simulink model "Acquisition_from_autosave"  (R2017a)
settings: Solver=VariableStepAuto  StartTime=0.0  StopTime=0.5  RelTol=1e-3
undefined symbols (not defined in the file): magnitude, Radix
libraries: simulink x34, commfilt2 x30, dspswit3 x12, dspmtrx3 x12, dspxfrm3 x3, simulink_extras x2, dspbuff3 x1
(part 2 of 4)

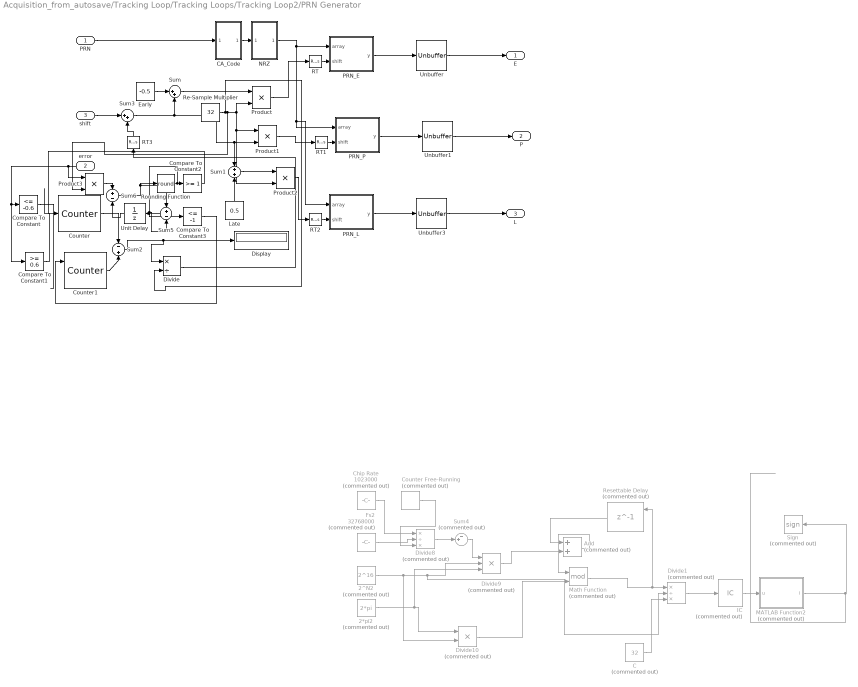
== system Acquisition_from_autosave/Tracking Loop/Tracking Loops/Tracking Loop2/PRN Generator  ==
  PRN : Inport
  error : Inport  Port=2  SampleTime=0.001
  shift : Inport  Port=3
  2*pi2 : Constant  Commented=on  Value=2*pi
  2^N2 : Constant  Commented=on  Value=2^16
  Add : Sum  Commented=on
  C : Constant  Commented=on  Value=32
  "CA_Code " : Subsystem
  Chip Rate : Constant  Commented=on  Value=1023000
  Compare To Constant : simulink/Logic and Bit Operations/Compare To Constant  relop=<=  const=-0.6  OutDataTypeStr=boolean
  Compare To Constant1 : simulink/Logic and Bit Operations/Compare To Constant  relop=>=  const=0.6  OutDataTypeStr=boolean
  Compare To Constant2 : simulink/Logic and Bit Operations/Compare To Constant  relop=>=  const=1  OutDataTypeStr=uint8
  Compare To Constant3 : simulink/Logic and Bit Operations/Compare To Constant  relop=<=  const=-1  OutDataTypeStr=uint8
  Counter : dspswit3/Counter  Direction=Up  CountEvent=Non-zero sample  CounterSize=User defined  MaxCount=255  InitialCount=0  Output=Count  HitValue=32  ResetInput=off  SamplesPerFrame=1  Ts=1  CntDtype=double  HitDtype=Logical
  Counter Free-Running : simulink/Sources/Counter Free-Running  Commented=on  NumBits=15  tsamp=1/32768000
  Counter1 : dspswit3/Counter  Direction=Up  CountEvent=Non-zero sample  CounterSize=User defined  MaxCount=255  InitialCount=0  Output=Count  HitValue=32  ResetInput=on  SamplesPerFrame=1  Ts=1  CntDtype=double  HitDtype=Logical
  Display : Display
  Divide : Product  Inputs=*/
  Divide1 : Product  Commented=on  Inputs=*/*
  Divide10 : Product  Commented=on
  Divide8 : Product  Commented=on  Inputs=*/*
  Divide9 : Product  Commented=on  Inputs=***
  Early : Constant  Value=-0.5
  Fs2 : Constant  Commented=on  Value=32768000
  IC : InitialCondition  Commented=on  Value=1023000
  Late : Constant  Value=0.5
  MATLAB Function2 : MATLAB Function  Commented=on  TreatAsAtomicUnit=on
  Math Function : Math  Commented=on  Operator=mod  SaturateOnIntegerOverflow=on
  NRZ : Subsystem
  PRN_E : MATLAB Function  TreatAsAtomicUnit=on  SystemSampleTime=0.001
  PRN_L : MATLAB Function  TreatAsAtomicUnit=on  SystemSampleTime=0.001
  PRN_P : MATLAB Function  TreatAsAtomicUnit=on  SystemSampleTime=0.001
  Product{,1..3} (4 alike) : Product
  RT : RateTransition  OutPortSampleTime=0.001
  RT1 : RateTransition  OutPortSampleTime=0.001
  RT2 : RateTransition  OutPortSampleTime=0.001
  RT3 : RateTransition
  Re-Sample Multiplier : Constant  Value=32
  Resettable Delay : Delay  Commented=on  DelayLength=1  ExternalReset=Rising  SampleTime=0.001
      settings: InputPortMap=u0,r5
  Rounding Function : Rounding  Operator=round
  Sign : Signum  Commented=on
  Sum : Sum  Inputs=|++
  Sum1 : Sum
  Sum2 : Sum  Inputs=-+
  Sum3 : Sum  Inputs=|++
  Sum4 : Sum  Commented=on  Inputs=-+|
  Sum5 : Sum  Inputs=+-
  Sum6 : Sum  Inputs=+-
  Unbuffer : Unbuffer
  Unbuffer1 : Unbuffer
  Unbuffer3 : Unbuffer
  Unit Delay : UnitDelay  SampleTime=0.001
  E : Outport
  P : Outport  Port=2
  L : Outport  Port=3
  wires:
  Product/1 -> RT/1
  PRN_E/1(y) -> Unbuffer/1
  Product2/1 -> RT2/1
  PRN_L/1(y) -> Unbuffer3/1
  Re-Sample Multiplier/1 -> Divide/2, Product3/2, Product1/1, Product2/2, Product/2
  PRN/1 -> "CA_Code "/1(In1)
  Unbuffer1/1 -> P/1
  Unbuffer3/1 -> L/1
  Early/1 -> Sum/1
  Sum/1 -> Product/1
  Sum3/1 -> Product1/2, Sum1/1, Sum/2
  Sum1/1 -> Product2/1
  PRN_P/1(y) -> Unbuffer1/1
  error/1 -> Product3/1, Compare To Constant1/1, Compare To Constant/1
  Counter/1 -> Sum2/1
  Counter1/1 -> Sum2/2
  Sum2/1 -> Divide/1, Display/1
  shift/1 -> Sum3/1
  RT/1 -> PRN_E/2(shift)
  RT1/1 -> PRN_P/2(shift)
  RT2/1 -> PRN_L/2(shift)
  Late/1 -> Sum1/2
  "CA_Code "/1(Out1) -> NRZ/1(In1)
  Unbuffer/1 -> E/1
  NRZ/1(Out1) -> PRN_E/1(array), PRN_L/1(array), PRN_P/1(array)
  Product1/1 -> RT1/1
  RT3/1 -> Sum3/2
  Compare To Constant1/1 -> ?
  Compare To Constant/1 -> ?
  MATLAB Function2/1(I) -> Sign/1
  Divide8/1 -> Sum4/2
  C/1 -> Divide1/3
  2^N2/1 -> Divide10/2, Divide1/2, Divide9/2
  Fs2/1 -> Divide8/2
  2*pi2/1 -> Divide9/3, Divide10/1
  Sum4/1 -> Divide9/1
  IC/1 -> MATLAB Function2/1(u)
  Divide10/1 -> Math Function/2
  Chip Rate/1 -> Divide8/1
  Resettable Delay/1 -> Add/1
  Divide1/1 -> IC/1
  Divide9/1 -> Add/2
  Counter Free-Running/1 -> Divide8/3
  Add/1 -> Math Function/1
  Math Function/1 -> Resettable Delay/1, Divide1/1
  Compare To Constant2/1 -> Counter/1
  Compare To Constant3/1 -> Counter1/1
  Divide/1 -> RT3/1
  Rounding Function/1 -> Sum5/2, Compare To Constant3/1, Compare To Constant2/1
  Product3/1 -> Sum6/1
  Sum5/1 -> Unit Delay/1
  Sum6/1 -> Sum5/1, Rounding Function/1
  Unit Delay/1 -> Sum6/2

== system Acquisition_from_autosave/Tracking Loop/Tracking Loops/Tracking Loop3/Carrier Filter ==
  In2 : Inport
  Add : Sum
  Constant : Constant  Value=0.001
  Constant1 : Constant  Value=-1
  Constant2 : Constant
  Constant3 : Constant  Value=-1
  Delay : Delay  DelayLength=1  InitialCondition=0  SampleTime=0.001
  Discrete FIR Filter : DiscreteFir  CoefSource=Input port  Coefficients=[2 1]  SampleTime=0.001
      settings: InputPortMap=u0,u1
  Discrete Filter : DiscreteFilter  NumeratorSource=Input port  DenominatorSource=Input port  SampleTime=0.001  a0EqualsOne=on
      settings: InputPortMap=u0,p1,p3
  Filter Parameters : Subsystem
  Product{,2..4} (4 alike) : Product
  Product1 : Product  Inputs=3
  Subsystem : Subsystem
  Sum : Sum  Inputs=|++
  Sum1 : Sum  Inputs=|++
  Sum3 : Sum  Inputs=|+-
  Sum4 : Sum  Inputs=+++
  Unit Delay : UnitDelay  SampleTime=0.001
  Unit Delay1 : UnitDelay  SampleTime=0.001
  Vector Concatenate : Concatenate
  Vector Concatenate1 : Concatenate
  Out1 : Outport
  wires:
  Product2/1 -> Sum/1
  Sum/1 -> Delay/1, Sum1/1
  Delay/1 -> Sum/2
  Product3/1 -> Sum1/2
  Unit Delay/1 -> Sum3/2
  Filter Parameters/1(K1) -> Product/2
  Filter Parameters/2(K2) -> Product1/2
  Constant/1 -> Product1/1
  Product1/1 -> Sum4/2
  Product/1 -> Sum4/1
  Sum4/1 -> Unit Delay1/1
  Unit Delay1/1 -> Sum4/3
  Subsystem/1("K2 ") -> Add/1, Product2/2
  Subsystem/2(K1) -> Product4/1, Add/2, Product3/1
  Sum3/1 -> Unit Delay/1, Product/1
  In2/1 -> Discrete Filter/1, Discrete FIR Filter/1, Product3/2, Product2/1
  ? -> Product1/3, Sum3/1
  Vector Concatenate/1 -> Discrete Filter/2, Discrete FIR Filter/2
  Constant1/1 -> Product4/2
  Product4/1 -> Vector Concatenate/2
  Add/1 -> Vector Concatenate/1
  Discrete Filter/1 -> Out1/1
  Constant2/1 -> Vector Concatenate1/1
  Constant3/1 -> Vector Concatenate1/2
  Vector Concatenate1/1 -> Discrete Filter/3

== system Acquisition_from_autosave/Tracking Loop/Tracking Loops/Tracking Loop3/Carrier Loop Discriminator  ==
  I_P : Inport
  Q_P : Inport  Port=2
  Constant : Constant  Value=2*pi
  Divide : Product  Inputs=/*
  Divide1 : Product  Inputs=*/
  IC : InitialCondition  Value=0
  IC1 : InitialCondition
  IC2 : InitialCondition
  atan : Trigonometry  Operator=atan
  theta : Outport
  wires:
  atan/1 -> Divide1/1
  Divide/1 -> atan/1
  I_P/1 -> IC1/1
  IC/1 -> theta/1
  Constant/1 -> Divide1/2
  Divide1/1 -> IC/1
  Q_P/1 -> IC2/1
  IC1/1 -> Divide/1
  IC2/1 -> Divide/2

== system Acquisition_from_autosave/Tracking Loop/Tracking Loops/Tracking Loop3/Code Filter ==
  In1 : Inport  SampleTime=0.001
  Add : Sum
  BW : Constant  Value=25
  Coeffiecients : Subsystem
  Constant : Constant  Value=2*pi
  Delay : Delay  DelayLength=1  InitialCondition=0  SampleTime=0.001
  Delay1 : Delay  DelayLength=1  InitialCondition=0  SampleTime=0.001
  Display : Display
  Display1 : Display
  Divide : Product  Inputs=*/
  Divide1 : Product  Inputs=**
  Divide2 : Product  Inputs=**
  Subtract : Sum  Inputs=-++
  ts : Constant  Value=0.001
  zeta : Constant  Value=0.7
  Out1 : Outport
  wires:
  Constant/1 -> Divide/2
  Divide/1 -> Delay/1, Divide2/1
  BW/1 -> Coeffiecients/1(BW)
  zeta/1 -> Coeffiecients/2(Zeta)
  ts/1 -> Coeffiecients/3(ts)
  Coeffiecients/1(C1) -> Add/1, Divide1/2
  Delay/1 -> Divide1/1
  Coeffiecients/2(C2) -> Add/2
  Add/1 -> Divide2/2
  Divide1/1 -> Subtract/1
  Divide2/1 -> Subtract/2
  Subtract/1 -> Out1/1, Delay1/1
  Delay1/1 -> Subtract/3
  In1/1 -> Divide/1

== system Acquisition_from_autosave/Tracking Loop/Tracking Loops/Tracking Loop3/Code Loop Discriminator ==
  I_E : Inport
  I_L : Inport  Port=2
  Q_E : Inport  Port=3
  Q_L : Inport  Port=4
  Add : Sum
  Add1 : Sum
  Add2 : Sum  Inputs=+-
  Add3 : Sum
  Display : Display
  Divide : Product  Inputs=*/
  IC : InitialCondition  Value=0
  Math Function{,2..3,5} (4 alike) : Math  Operator=magnitude^2  RndMeth=Zero  SaturateOnIntegerOverflow=on
  Sqrt : Sqrt  SaturateOnIntegerOverflow=on
  Sqrt1 : Sqrt  SaturateOnIntegerOverflow=on
  error : Outport
  wires:
  I_L/1 -> Math Function2/1
  I_E/1 -> Math Function/1
  Q_E/1 -> Math Function3/1
  Q_L/1 -> Math Function5/1
  Math Function2/1 -> Add1/1
  Math Function5/1 -> Add1/2
  Math Function/1 -> Add/1
  Math Function3/1 -> Add/2
  Add2/1 -> Divide/1
  Add3/1 -> Divide/2
  Divide/1 -> IC/1
  IC/1 -> Display/1, error/1
  Add/1 -> Sqrt/1
  Add1/1 -> Sqrt1/1
  Sqrt/1 -> Add3/1, Add2/1
  Sqrt1/1 -> Add3/2, Add2/2

== system Acquisition_from_autosave/Tracking Loop/Tracking Loops/Tracking Loop3/Controlled Carrier Generator ==
  Freq ACQ : Inport
  Phase Error : Inport  Port=2
  Freq Error : Inport  Port=3
  Clock : Clock  Commented=on
  Clock1 : Clock
  Discrete Derivative : simulink/Discrete/Discrete Derivative  gainval=1.0  ICPrevScaledInput=0.0  OutMin=[]  OutMax=[]  OutDataType=fixdt(1, 16)  OutScaling=2^-10  DoSatur=off
  Display : Display
  MATLAB Function : MATLAB Function  TreatAsAtomicUnit=on
  MATLAB Function1 : MATLAB Function  Commented=on  TreatAsAtomicUnit=on
  Sum : Sum  Inputs=++|
  "wave " : Outport
  wires:
  Clock/1 -> MATLAB Function1/2(timer)
  Freq Error/1 -> Sum/1
  Freq ACQ/1 -> Sum/2
  Sum/1 -> MATLAB Function/2(freq)
  Clock1/1 -> MATLAB Function/1(time)
  Phase Error/1 -> Discrete Derivative/1, MATLAB Function/3(phase)
  MATLAB Function/1(wave) -> "wave "/1
  Discrete Derivative/1 -> Display/1

== system Acquisition_from_autosave/Tracking Loop/Tracking Loops/Tracking Loop3/Oscillator ==
  phase error : Inport
  Acq Freq : Inport  Port=2
  2*pi2 : Constant  Value=2*pi
  2^N2 : Constant  Value=2^16
  Add : Sum
  Counter Free-Running : simulink/Sources/Counter Free-Running  NumBits=15  tsamp=1/32768000
  Divide1 : Product  Inputs=*/
  Divide10 : Product
  Divide8 : Product  Inputs=*/*
  Divide9 : Product  Inputs=***
  Fs2 : Constant  Value=32768000
  IC : InitialCondition  Value=9207000
  MATLAB Function2 : MATLAB Function  TreatAsAtomicUnit=on
  Math Function : Math  Operator=mod  SaturateOnIntegerOverflow=on
  Pulse Generator1 : DiscretePulseGenerator  PulseType=Time based  Period=0.005  PulseWidth=50
  RT2 : RateTransition
  Real-Imag to Complex2 : RealImagToComplex
  Resettable Delay : Delay  DelayLength=1  ExternalReset=Rising  SampleTime=0.001
      settings: InputPortMap=u0,r5
  Sum2 : Sum  Inputs=-+|
  Out1 : Outport
  wires:
  2*pi2/1 -> Divide9/3, Divide10/1
  Sum2/1 -> Divide9/1
  Divide8/1 -> Sum2/2
  2^N2/1 -> Divide10/2, Divide1/2, Divide9/2
  Fs2/1 -> Divide8/2
  Divide10/1 -> Math Function/2
  phase error/1 -> Sum2/1
  Acq Freq/1 -> Divide8/1
  Pulse Generator1/1 -> RT2/1
  MATLAB Function2/1(I) -> Real-Imag to Complex2/1
  MATLAB Function2/2(Q) -> Real-Imag to Complex2/2
  Divide1/1 -> IC/1
  IC/1 -> MATLAB Function2/1(u)
  Resettable Delay/1 -> Add/1
  Math Function/1 -> Resettable Delay/1, Divide1/1
  Add/1 -> Math Function/1
  Divide9/1 -> Add/2
  Real-Imag to Complex2/1 -> Out1/1
  Counter Free-Running/1 -> Divide8/3

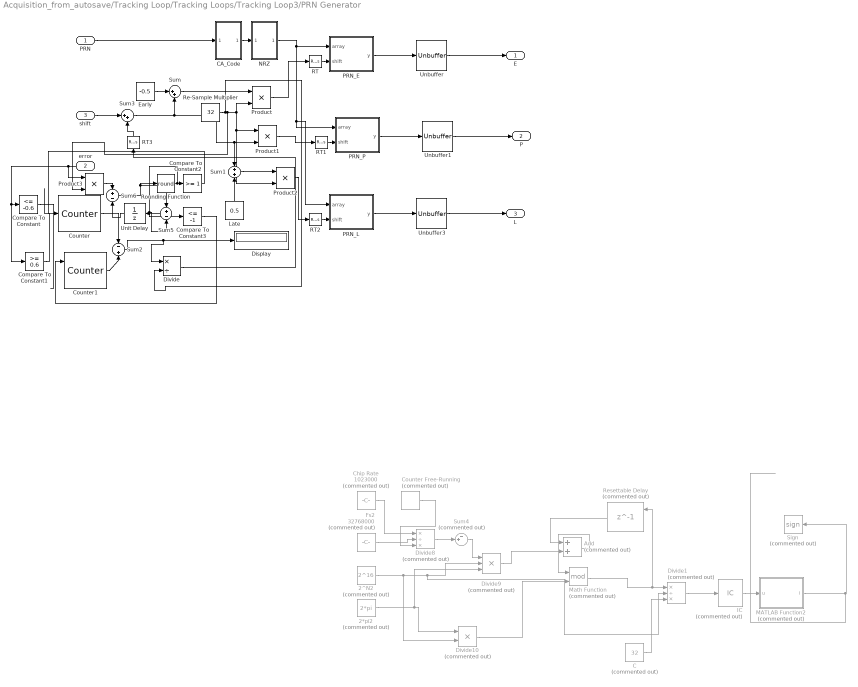
== system Acquisition_from_autosave/Tracking Loop/Tracking Loops/Tracking Loop3/PRN Generator  ==
  PRN : Inport
  error : Inport  Port=2  SampleTime=0.001
  shift : Inport  Port=3
  2*pi2 : Constant  Commented=on  Value=2*pi
  2^N2 : Constant  Commented=on  Value=2^16
  Add : Sum  Commented=on
  C : Constant  Commented=on  Value=32
  "CA_Code " : Subsystem
  Chip Rate : Constant  Commented=on  Value=1023000
  Compare To Constant : simulink/Logic and Bit Operations/Compare To Constant  relop=<=  const=-0.6  OutDataTypeStr=boolean
  Compare To Constant1 : simulink/Logic and Bit Operations/Compare To Constant  relop=>=  const=0.6  OutDataTypeStr=boolean
  Compare To Constant2 : simulink/Logic and Bit Operations/Compare To Constant  relop=>=  const=1  OutDataTypeStr=uint8
  Compare To Constant3 : simulink/Logic and Bit Operations/Compare To Constant  relop=<=  const=-1  OutDataTypeStr=uint8
  Counter : dspswit3/Counter  Direction=Up  CountEvent=Non-zero sample  CounterSize=User defined  MaxCount=255  InitialCount=0  Output=Count  HitValue=32  ResetInput=off  SamplesPerFrame=1  Ts=1  CntDtype=double  HitDtype=Logical
  Counter Free-Running : simulink/Sources/Counter Free-Running  Commented=on  NumBits=15  tsamp=1/32768000
  Counter1 : dspswit3/Counter  Direction=Up  CountEvent=Non-zero sample  CounterSize=User defined  MaxCount=255  InitialCount=0  Output=Count  HitValue=32  ResetInput=on  SamplesPerFrame=1  Ts=1  CntDtype=double  HitDtype=Logical
  Display : Display
  Divide : Product  Inputs=*/
  Divide1 : Product  Commented=on  Inputs=*/*
  Divide10 : Product  Commented=on
  Divide8 : Product  Commented=on  Inputs=*/*
  Divide9 : Product  Commented=on  Inputs=***
  Early : Constant  Value=-0.5
  Fs2 : Constant  Commented=on  Value=32768000
  IC : InitialCondition  Commented=on  Value=1023000
  Late : Constant  Value=0.5
  MATLAB Function2 : MATLAB Function  Commented=on  TreatAsAtomicUnit=on
  Math Function : Math  Commented=on  Operator=mod  SaturateOnIntegerOverflow=on
  NRZ : Subsystem
  PRN_E : MATLAB Function  TreatAsAtomicUnit=on  SystemSampleTime=0.001
  PRN_L : MATLAB Function  TreatAsAtomicUnit=on  SystemSampleTime=0.001
  PRN_P : MATLAB Function  TreatAsAtomicUnit=on  SystemSampleTime=0.001
  Product{,1..3} (4 alike) : Product
  RT : RateTransition  OutPortSampleTime=0.001
  RT1 : RateTransition  OutPortSampleTime=0.001
  RT2 : RateTransition  OutPortSampleTime=0.001
  RT3 : RateTransition
  Re-Sample Multiplier : Constant  Value=32
  Resettable Delay : Delay  Commented=on  DelayLength=1  ExternalReset=Rising  SampleTime=0.001
      settings: InputPortMap=u0,r5
  Rounding Function : Rounding  Operator=round
  Sign : Signum  Commented=on
  Sum : Sum  Inputs=|++
  Sum1 : Sum
  Sum2 : Sum  Inputs=-+
  Sum3 : Sum  Inputs=|++
  Sum4 : Sum  Commented=on  Inputs=-+|
  Sum5 : Sum  Inputs=+-
  Sum6 : Sum  Inputs=+-
  Unbuffer : Unbuffer
  Unbuffer1 : Unbuffer
  Unbuffer3 : Unbuffer
  Unit Delay : UnitDelay  SampleTime=0.001
  E : Outport
  P : Outport  Port=2
  L : Outport  Port=3
  wires:
  Product/1 -> RT/1
  PRN_E/1(y) -> Unbuffer/1
  Product2/1 -> RT2/1
  PRN_L/1(y) -> Unbuffer3/1
  Re-Sample Multiplier/1 -> Divide/2, Product3/2, Product1/1, Product2/2, Product/2
  PRN/1 -> "CA_Code "/1(In1)
  Unbuffer1/1 -> P/1
  Unbuffer3/1 -> L/1
  Early/1 -> Sum/1
  Sum/1 -> Product/1
  Sum3/1 -> Product1/2, Sum1/1, Sum/2
  Sum1/1 -> Product2/1
  PRN_P/1(y) -> Unbuffer1/1
  error/1 -> Product3/1, Compare To Constant1/1, Compare To Constant/1
  Counter/1 -> Sum2/1
  Counter1/1 -> Sum2/2
  Sum2/1 -> Divide/1, Display/1
  shift/1 -> Sum3/1
  RT/1 -> PRN_E/2(shift)
  RT1/1 -> PRN_P/2(shift)
  RT2/1 -> PRN_L/2(shift)
  Late/1 -> Sum1/2
  "CA_Code "/1(Out1) -> NRZ/1(In1)
  Unbuffer/1 -> E/1
  NRZ/1(Out1) -> PRN_E/1(array), PRN_L/1(array), PRN_P/1(array)
  Product1/1 -> RT1/1
  RT3/1 -> Sum3/2
  Compare To Constant1/1 -> ?
  Compare To Constant/1 -> ?
  MATLAB Function2/1(I) -> Sign/1
  Divide8/1 -> Sum4/2
  C/1 -> Divide1/3
  2^N2/1 -> Divide10/2, Divide1/2, Divide9/2
  Fs2/1 -> Divide8/2
  2*pi2/1 -> Divide9/3, Divide10/1
  Sum4/1 -> Divide9/1
  IC/1 -> MATLAB Function2/1(u)
  Divide10/1 -> Math Function/2
  Chip Rate/1 -> Divide8/1
  Resettable Delay/1 -> Add/1
  Divide1/1 -> IC/1
  Divide9/1 -> Add/2
  Counter Free-Running/1 -> Divide8/3
  Add/1 -> Math Function/1
  Math Function/1 -> Resettable Delay/1, Divide1/1
  Compare To Constant2/1 -> Counter/1
  Compare To Constant3/1 -> Counter1/1
  Divide/1 -> RT3/1
  Rounding Function/1 -> Sum5/2, Compare To Constant3/1, Compare To Constant2/1
  Product3/1 -> Sum6/1
  Sum5/1 -> Unit Delay/1
  Sum6/1 -> Sum5/1, Rounding Function/1
  Unit Delay/1 -> Sum6/2

== system Acquisition_from_autosave/Tracking Loop/Tracking Loops/Tracking Loop4/Carrier Filter ==
  In2 : Inport
  Add : Sum
  Constant : Constant  Value=0.001
  Constant1 : Constant  Value=-1
  Constant2 : Constant
  Constant3 : Constant  Value=-1
  Delay : Delay  DelayLength=1  InitialCondition=0  SampleTime=0.001
  Discrete FIR Filter : DiscreteFir  CoefSource=Input port  Coefficients=[2 1]  SampleTime=0.001
      settings: InputPortMap=u0,u1
  Discrete Filter : DiscreteFilter  NumeratorSource=Input port  DenominatorSource=Input port  SampleTime=0.001  a0EqualsOne=on
      settings: InputPortMap=u0,p1,p3
  Filter Parameters : Subsystem
  Product{,2..4} (4 alike) : Product
  Product1 : Product  Inputs=3
  Subsystem : Subsystem
  Sum : Sum  Inputs=|++
  Sum1 : Sum  Inputs=|++
  Sum3 : Sum  Inputs=|+-
  Sum4 : Sum  Inputs=+++
  Unit Delay : UnitDelay  SampleTime=0.001
  Unit Delay1 : UnitDelay  SampleTime=0.001
  Vector Concatenate : Concatenate
  Vector Concatenate1 : Concatenate
  Out1 : Outport
  wires:
  Product2/1 -> Sum/1
  Sum/1 -> Delay/1, Sum1/1
  Delay/1 -> Sum/2
  Product3/1 -> Sum1/2
  Unit Delay/1 -> Sum3/2
  Filter Parameters/1(K1) -> Product/2
  Filter Parameters/2(K2) -> Product1/2
  Constant/1 -> Product1/1
  Product1/1 -> Sum4/2
  Product/1 -> Sum4/1
  Sum4/1 -> Unit Delay1/1
  Unit Delay1/1 -> Sum4/3
  Subsystem/1("K2 ") -> Add/1, Product2/2
  Subsystem/2(K1) -> Product4/1, Add/2, Product3/1
  Sum3/1 -> Unit Delay/1, Product/1
  In2/1 -> Discrete Filter/1, Discrete FIR Filter/1, Product3/2, Product2/1
  ? -> Product1/3, Sum3/1
  Vector Concatenate/1 -> Discrete Filter/2, Discrete FIR Filter/2
  Constant1/1 -> Product4/2
  Product4/1 -> Vector Concatenate/2
  Add/1 -> Vector Concatenate/1
  Discrete Filter/1 -> Out1/1
  Constant2/1 -> Vector Concatenate1/1
  Constant3/1 -> Vector Concatenate1/2
  Vector Concatenate1/1 -> Discrete Filter/3

== system Acquisition_from_autosave/Tracking Loop/Tracking Loops/Tracking Loop4/Carrier Loop Discriminator  ==
  I_P : Inport
  Q_P : Inport  Port=2
  Constant : Constant  Value=2*pi
  Divide : Product  Inputs=/*
  Divide1 : Product  Inputs=*/
  IC : InitialCondition  Value=0
  IC1 : InitialCondition
  IC2 : InitialCondition
  atan : Trigonometry  Operator=atan
  theta : Outport
  wires:
  atan/1 -> Divide1/1
  Divide/1 -> atan/1
  I_P/1 -> IC1/1
  IC/1 -> theta/1
  Constant/1 -> Divide1/2
  Divide1/1 -> IC/1
  Q_P/1 -> IC2/1
  IC1/1 -> Divide/1
  IC2/1 -> Divide/2

== system Acquisition_from_autosave/Tracking Loop/Tracking Loops/Tracking Loop4/Code Filter ==
  In1 : Inport  SampleTime=0.001
  Add : Sum
  BW : Constant  Value=25
  Coeffiecients : Subsystem
  Constant : Constant  Value=2*pi
  Delay : Delay  DelayLength=1  InitialCondition=0  SampleTime=0.001
  Delay1 : Delay  DelayLength=1  InitialCondition=0  SampleTime=0.001
  Display : Display
  Display1 : Display
  Divide : Product  Inputs=*/
  Divide1 : Product  Inputs=**
  Divide2 : Product  Inputs=**
  Subtract : Sum  Inputs=-++
  ts : Constant  Value=0.001
  zeta : Constant  Value=0.7
  Out1 : Outport
  wires:
  Constant/1 -> Divide/2
  Divide/1 -> Delay/1, Divide2/1
  BW/1 -> Coeffiecients/1(BW)
  zeta/1 -> Coeffiecients/2(Zeta)
  ts/1 -> Coeffiecients/3(ts)
  Coeffiecients/1(C1) -> Add/1, Divide1/2
  Delay/1 -> Divide1/1
  Coeffiecients/2(C2) -> Add/2
  Add/1 -> Divide2/2
  Divide1/1 -> Subtract/1
  Divide2/1 -> Subtract/2
  Subtract/1 -> Out1/1, Delay1/1
  Delay1/1 -> Subtract/3
  In1/1 -> Divide/1

== system Acquisition_from_autosave/Tracking Loop/Tracking Loops/Tracking Loop4/Code Loop Discriminator ==
  I_E : Inport
  I_L : Inport  Port=2
  Q_E : Inport  Port=3
  Q_L : Inport  Port=4
  Add : Sum
  Add1 : Sum
  Add2 : Sum  Inputs=+-
  Add3 : Sum
  Display : Display
  Divide : Product  Inputs=*/
  IC : InitialCondition  Value=0
  Math Function{,2..3,5} (4 alike) : Math  Operator=magnitude^2  RndMeth=Zero  SaturateOnIntegerOverflow=on
  Sqrt : Sqrt  SaturateOnIntegerOverflow=on
  Sqrt1 : Sqrt  SaturateOnIntegerOverflow=on
  error : Outport
  wires:
  I_L/1 -> Math Function2/1
  I_E/1 -> Math Function/1
  Q_E/1 -> Math Function3/1
  Q_L/1 -> Math Function5/1
  Math Function2/1 -> Add1/1
  Math Function5/1 -> Add1/2
  Math Function/1 -> Add/1
  Math Function3/1 -> Add/2
  Add2/1 -> Divide/1
  Add3/1 -> Divide/2
  Divide/1 -> IC/1
  IC/1 -> Display/1, error/1
  Add/1 -> Sqrt/1
  Add1/1 -> Sqrt1/1
  Sqrt/1 -> Add3/1, Add2/1
  Sqrt1/1 -> Add3/2, Add2/2

== system Acquisition_from_autosave/Tracking Loop/Tracking Loops/Tracking Loop4/Controlled Carrier Generator ==
  Freq ACQ : Inport
  Phase Error : Inport  Port=2
  Freq Error : Inport  Port=3
  Clock : Clock  Commented=on
  Clock1 : Clock
  Discrete Derivative : simulink/Discrete/Discrete Derivative  gainval=1.0  ICPrevScaledInput=0.0  OutMin=[]  OutMax=[]  OutDataType=fixdt(1, 16)  OutScaling=2^-10  DoSatur=off
  Display : Display
  MATLAB Function : MATLAB Function  TreatAsAtomicUnit=on
  MATLAB Function1 : MATLAB Function  Commented=on  TreatAsAtomicUnit=on
  Sum : Sum  Inputs=++|
  "wave " : Outport
  wires:
  Clock/1 -> MATLAB Function1/2(timer)
  Freq Error/1 -> Sum/1
  Freq ACQ/1 -> Sum/2
  Sum/1 -> MATLAB Function/2(freq)
  Clock1/1 -> MATLAB Function/1(time)
  Phase Error/1 -> Discrete Derivative/1, MATLAB Function/3(phase)
  MATLAB Function/1(wave) -> "wave "/1
  Discrete Derivative/1 -> Display/1

== system Acquisition_from_autosave/Tracking Loop/Tracking Loops/Tracking Loop4/Oscillator ==
  phase error : Inport
  Acq Freq : Inport  Port=2
  2*pi2 : Constant  Value=2*pi
  2^N2 : Constant  Value=2^16
  Add : Sum
  Counter Free-Running : simulink/Sources/Counter Free-Running  NumBits=15  tsamp=1/32768000
  Divide1 : Product  Inputs=*/
  Divide10 : Product
  Divide8 : Product  Inputs=*/*
  Divide9 : Product  Inputs=***
  Fs2 : Constant  Value=32768000
  IC : InitialCondition  Value=9207000
  MATLAB Function2 : MATLAB Function  TreatAsAtomicUnit=on
  Math Function : Math  Operator=mod  SaturateOnIntegerOverflow=on
  Pulse Generator1 : DiscretePulseGenerator  PulseType=Time based  Period=0.005  PulseWidth=50
  RT2 : RateTransition
  Real-Imag to Complex2 : RealImagToComplex
  Resettable Delay : Delay  DelayLength=1  ExternalReset=Rising  SampleTime=0.001
      settings: InputPortMap=u0,r5
  Sum2 : Sum  Inputs=-+|
  Out1 : Outport
  wires:
  2*pi2/1 -> Divide9/3, Divide10/1
  Sum2/1 -> Divide9/1
  Divide8/1 -> Sum2/2
  2^N2/1 -> Divide10/2, Divide1/2, Divide9/2
  Fs2/1 -> Divide8/2
  Divide10/1 -> Math Function/2
  phase error/1 -> Sum2/1
  Acq Freq/1 -> Divide8/1
  Pulse Generator1/1 -> RT2/1
  MATLAB Function2/1(I) -> Real-Imag to Complex2/1
  MATLAB Function2/2(Q) -> Real-Imag to Complex2/2
  Divide1/1 -> IC/1
  IC/1 -> MATLAB Function2/1(u)
  Resettable Delay/1 -> Add/1
  Math Function/1 -> Resettable Delay/1, Divide1/1
  Add/1 -> Math Function/1
  Divide9/1 -> Add/2
  Real-Imag to Complex2/1 -> Out1/1
  Counter Free-Running/1 -> Divide8/3

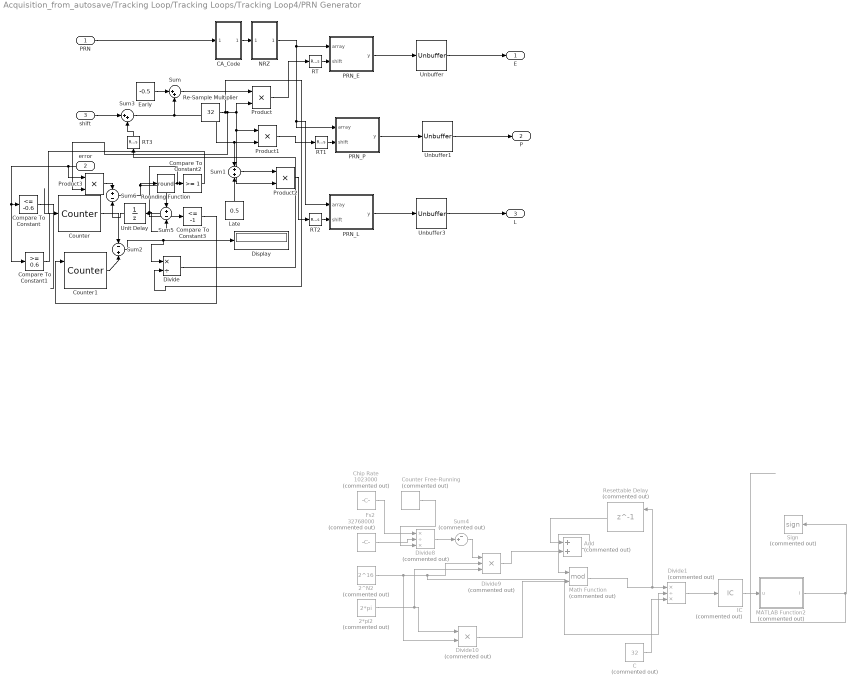
== system Acquisition_from_autosave/Tracking Loop/Tracking Loops/Tracking Loop4/PRN Generator  ==
  PRN : Inport
  error : Inport  Port=2  SampleTime=0.001
  shift : Inport  Port=3
  2*pi2 : Constant  Commented=on  Value=2*pi
  2^N2 : Constant  Commented=on  Value=2^16
  Add : Sum  Commented=on
  C : Constant  Commented=on  Value=32
  "CA_Code " : Subsystem
  Chip Rate : Constant  Commented=on  Value=1023000
  Compare To Constant : simulink/Logic and Bit Operations/Compare To Constant  relop=<=  const=-0.6  OutDataTypeStr=boolean
  Compare To Constant1 : simulink/Logic and Bit Operations/Compare To Constant  relop=>=  const=0.6  OutDataTypeStr=boolean
  Compare To Constant2 : simulink/Logic and Bit Operations/Compare To Constant  relop=>=  const=1  OutDataTypeStr=uint8
  Compare To Constant3 : simulink/Logic and Bit Operations/Compare To Constant  relop=<=  const=-1  OutDataTypeStr=uint8
  Counter : dspswit3/Counter  Direction=Up  CountEvent=Non-zero sample  CounterSize=User defined  MaxCount=255  InitialCount=0  Output=Count  HitValue=32  ResetInput=off  SamplesPerFrame=1  Ts=1  CntDtype=double  HitDtype=Logical
  Counter Free-Running : simulink/Sources/Counter Free-Running  Commented=on  NumBits=15  tsamp=1/32768000
  Counter1 : dspswit3/Counter  Direction=Up  CountEvent=Non-zero sample  CounterSize=User defined  MaxCount=255  InitialCount=0  Output=Count  HitValue=32  ResetInput=on  SamplesPerFrame=1  Ts=1  CntDtype=double  HitDtype=Logical
  Display : Display
  Divide : Product  Inputs=*/
  Divide1 : Product  Commented=on  Inputs=*/*
  Divide10 : Product  Commented=on
  Divide8 : Product  Commented=on  Inputs=*/*
  Divide9 : Product  Commented=on  Inputs=***
  Early : Constant  Value=-0.5
  Fs2 : Constant  Commented=on  Value=32768000
  IC : InitialCondition  Commented=on  Value=1023000
  Late : Constant  Value=0.5
  MATLAB Function2 : MATLAB Function  Commented=on  TreatAsAtomicUnit=on
  Math Function : Math  Commented=on  Operator=mod  SaturateOnIntegerOverflow=on
  NRZ : Subsystem
  PRN_E : MATLAB Function  TreatAsAtomicUnit=on  SystemSampleTime=0.001
  PRN_L : MATLAB Function  TreatAsAtomicUnit=on  SystemSampleTime=0.001
  PRN_P : MATLAB Function  TreatAsAtomicUnit=on  SystemSampleTime=0.001
  Product{,1..3} (4 alike) : Product
  RT : RateTransition  OutPortSampleTime=0.001
  RT1 : RateTransition  OutPortSampleTime=0.001
  RT2 : RateTransition  OutPortSampleTime=0.001
  RT3 : RateTransition
  Re-Sample Multiplier : Constant  Value=32
  Resettable Delay : Delay  Commented=on  DelayLength=1  ExternalReset=Rising  SampleTime=0.001
      settings: InputPortMap=u0,r5
  Rounding Function : Rounding  Operator=round
  Sign : Signum  Commented=on
  Sum : Sum  Inputs=|++
  Sum1 : Sum
  Sum2 : Sum  Inputs=-+
  Sum3 : Sum  Inputs=|++
  Sum4 : Sum  Commented=on  Inputs=-+|
  Sum5 : Sum  Inputs=+-
  Sum6 : Sum  Inputs=+-
  Unbuffer : Unbuffer
  Unbuffer1 : Unbuffer
  Unbuffer3 : Unbuffer
  Unit Delay : UnitDelay  SampleTime=0.001
  E : Outport
  P : Outport  Port=2
  L : Outport  Port=3
  wires:
  Product/1 -> RT/1
  PRN_E/1(y) -> Unbuffer/1
  Product2/1 -> RT2/1
  PRN_L/1(y) -> Unbuffer3/1
  Re-Sample Multiplier/1 -> Divide/2, Product3/2, Product1/1, Product2/2, Product/2
  PRN/1 -> "CA_Code "/1(In1)
  Unbuffer1/1 -> P/1
  Unbuffer3/1 -> L/1
  Early/1 -> Sum/1
  Sum/1 -> Product/1
  Sum3/1 -> Product1/2, Sum1/1, Sum/2
  Sum1/1 -> Product2/1
  PRN_P/1(y) -> Unbuffer1/1
  error/1 -> Product3/1, Compare To Constant1/1, Compare To Constant/1
  Counter/1 -> Sum2/1
  Counter1/1 -> Sum2/2
  Sum2/1 -> Divide/1, Display/1
  shift/1 -> Sum3/1
  RT/1 -> PRN_E/2(shift)
  RT1/1 -> PRN_P/2(shift)
  RT2/1 -> PRN_L/2(shift)
  Late/1 -> Sum1/2
  "CA_Code "/1(Out1) -> NRZ/1(In1)
  Unbuffer/1 -> E/1
  NRZ/1(Out1) -> PRN_E/1(array), PRN_L/1(array), PRN_P/1(array)
  Product1/1 -> RT1/1
  RT3/1 -> Sum3/2
  Compare To Constant1/1 -> ?
  Compare To Constant/1 -> ?
  MATLAB Function2/1(I) -> Sign/1
  Divide8/1 -> Sum4/2
  C/1 -> Divide1/3
  2^N2/1 -> Divide10/2, Divide1/2, Divide9/2
  Fs2/1 -> Divide8/2
  2*pi2/1 -> Divide9/3, Divide10/1
  Sum4/1 -> Divide9/1
  IC/1 -> MATLAB Function2/1(u)
  Divide10/1 -> Math Function/2
  Chip Rate/1 -> Divide8/1
  Resettable Delay/1 -> Add/1
  Divide1/1 -> IC/1
  Divide9/1 -> Add/2
  Counter Free-Running/1 -> Divide8/3
  Add/1 -> Math Function/1
  Math Function/1 -> Resettable Delay/1, Divide1/1
  Compare To Constant2/1 -> Counter/1
  Compare To Constant3/1 -> Counter1/1
  Divide/1 -> RT3/1
  Rounding Function/1 -> Sum5/2, Compare To Constant3/1, Compare To Constant2/1
  Product3/1 -> Sum6/1
  Sum5/1 -> Unit Delay/1
  Sum6/1 -> Sum5/1, Rounding Function/1
  Unit Delay/1 -> Sum6/2

== system Acquisition_from_autosave/Tracking Loop/Tracking Loops/Tracking Loop5/Carrier Filter ==
  In2 : Inport
  Add : Sum
  Constant : Constant  Value=0.001
  Constant1 : Constant  Value=-1
  Constant2 : Constant
  Constant3 : Constant  Value=-1
  Delay : Delay  DelayLength=1  InitialCondition=0  SampleTime=0.001
  Discrete FIR Filter : DiscreteFir  CoefSource=Input port  Coefficients=[2 1]  SampleTime=0.001
      settings: InputPortMap=u0,u1
  Discrete Filter : DiscreteFilter  NumeratorSource=Input port  DenominatorSource=Input port  SampleTime=0.001  a0EqualsOne=on
      settings: InputPortMap=u0,p1,p3
  Filter Parameters : Subsystem
  Product{,2..4} (4 alike) : Product
  Product1 : Product  Inputs=3
  Subsystem : Subsystem
  Sum : Sum  Inputs=|++
  Sum1 : Sum  Inputs=|++
  Sum3 : Sum  Inputs=|+-
  Sum4 : Sum  Inputs=+++
  Unit Delay : UnitDelay  SampleTime=0.001
  Unit Delay1 : UnitDelay  SampleTime=0.001
  Vector Concatenate : Concatenate
  Vector Concatenate1 : Concatenate
  Out1 : Outport
  wires:
  Product2/1 -> Sum/1
  Sum/1 -> Delay/1, Sum1/1
  Delay/1 -> Sum/2
  Product3/1 -> Sum1/2
  Unit Delay/1 -> Sum3/2
  Filter Parameters/1(K1) -> Product/2
  Filter Parameters/2(K2) -> Product1/2
  Constant/1 -> Product1/1
  Product1/1 -> Sum4/2
  Product/1 -> Sum4/1
  Sum4/1 -> Unit Delay1/1
  Unit Delay1/1 -> Sum4/3
  Subsystem/1("K2 ") -> Add/1, Product2/2
  Subsystem/2(K1) -> Product4/1, Add/2, Product3/1
  Sum3/1 -> Unit Delay/1, Product/1
  In2/1 -> Discrete Filter/1, Discrete FIR Filter/1, Product3/2, Product2/1
  ? -> Product1/3, Sum3/1
  Vector Concatenate/1 -> Discrete Filter/2, Discrete FIR Filter/2
  Constant1/1 -> Product4/2
  Product4/1 -> Vector Concatenate/2
  Add/1 -> Vector Concatenate/1
  Discrete Filter/1 -> Out1/1
  Constant2/1 -> Vector Concatenate1/1
  Constant3/1 -> Vector Concatenate1/2
  Vector Concatenate1/1 -> Discrete Filter/3

== system Acquisition_from_autosave/Tracking Loop/Tracking Loops/Tracking Loop5/Carrier Loop Discriminator  ==
  I_P : Inport
  Q_P : Inport  Port=2
  Constant : Constant  Value=2*pi
  Divide : Product  Inputs=/*
  Divide1 : Product  Inputs=*/
  IC : InitialCondition  Value=0
  IC1 : InitialCondition
  IC2 : InitialCondition
  atan : Trigonometry  Operator=atan
  theta : Outport
  wires:
  atan/1 -> Divide1/1
  Divide/1 -> atan/1
  I_P/1 -> IC1/1
  IC/1 -> theta/1
  Constant/1 -> Divide1/2
  Divide1/1 -> IC/1
  Q_P/1 -> IC2/1
  IC1/1 -> Divide/1
  IC2/1 -> Divide/2

== system Acquisition_from_autosave/Tracking Loop/Tracking Loops/Tracking Loop5/Code Filter ==
  In1 : Inport  SampleTime=0.001
  Add : Sum
  BW : Constant  Value=25
  Coeffiecients : Subsystem
  Constant : Constant  Value=2*pi
  Delay : Delay  DelayLength=1  InitialCondition=0  SampleTime=0.001
  Delay1 : Delay  DelayLength=1  InitialCondition=0  SampleTime=0.001
  Display : Display
  Display1 : Display
  Divide : Product  Inputs=*/
  Divide1 : Product  Inputs=**
  Divide2 : Product  Inputs=**
  Subtract : Sum  Inputs=-++
  ts : Constant  Value=0.001
  zeta : Constant  Value=0.7
  Out1 : Outport
  wires:
  Constant/1 -> Divide/2
  Divide/1 -> Delay/1, Divide2/1
  BW/1 -> Coeffiecients/1(BW)
  zeta/1 -> Coeffiecients/2(Zeta)
  ts/1 -> Coeffiecients/3(ts)
  Coeffiecients/1(C1) -> Add/1, Divide1/2
  Delay/1 -> Divide1/1
  Coeffiecients/2(C2) -> Add/2
  Add/1 -> Divide2/2
  Divide1/1 -> Subtract/1
  Divide2/1 -> Subtract/2
  Subtract/1 -> Out1/1, Delay1/1
  Delay1/1 -> Subtract/3
  In1/1 -> Divide/1

== system Acquisition_from_autosave/Tracking Loop/Tracking Loops/Tracking Loop5/Code Loop Discriminator ==
  I_E : Inport
  I_L : Inport  Port=2
  Q_E : Inport  Port=3
  Q_L : Inport  Port=4
  Add : Sum
  Add1 : Sum
  Add2 : Sum  Inputs=+-
  Add3 : Sum
  Display : Display
  Divide : Product  Inputs=*/
  IC : InitialCondition  Value=0
  Math Function{,2..3,5} (4 alike) : Math  Operator=magnitude^2  RndMeth=Zero  SaturateOnIntegerOverflow=on
  Sqrt : Sqrt  SaturateOnIntegerOverflow=on
  Sqrt1 : Sqrt  SaturateOnIntegerOverflow=on
  error : Outport
  wires:
  I_L/1 -> Math Function2/1
  I_E/1 -> Math Function/1
  Q_E/1 -> Math Function3/1
  Q_L/1 -> Math Function5/1
  Math Function2/1 -> Add1/1
  Math Function5/1 -> Add1/2
  Math Function/1 -> Add/1
  Math Function3/1 -> Add/2
  Add2/1 -> Divide/1
  Add3/1 -> Divide/2
  Divide/1 -> IC/1
  IC/1 -> Display/1, error/1
  Add/1 -> Sqrt/1
  Add1/1 -> Sqrt1/1
  Sqrt/1 -> Add3/1, Add2/1
  Sqrt1/1 -> Add3/2, Add2/2

== system Acquisition_from_autosave/Tracking Loop/Tracking Loops/Tracking Loop5/Controlled Carrier Generator ==
  Freq ACQ : Inport
  Phase Error : Inport  Port=2
  Freq Error : Inport  Port=3
  Clock : Clock  Commented=on
  Clock1 : Clock
  Discrete Derivative : simulink/Discrete/Discrete Derivative  gainval=1.0  ICPrevScaledInput=0.0  OutMin=[]  OutMax=[]  OutDataType=fixdt(1, 16)  OutScaling=2^-10  DoSatur=off
  Display : Display
  MATLAB Function : MATLAB Function  TreatAsAtomicUnit=on
  MATLAB Function1 : MATLAB Function  Commented=on  TreatAsAtomicUnit=on
  Sum : Sum  Inputs=++|
  "wave " : Outport
  wires:
  Clock/1 -> MATLAB Function1/2(timer)
  Freq Error/1 -> Sum/1
  Freq ACQ/1 -> Sum/2
  Sum/1 -> MATLAB Function/2(freq)
  Clock1/1 -> MATLAB Function/1(time)
  Phase Error/1 -> Discrete Derivative/1, MATLAB Function/3(phase)
  MATLAB Function/1(wave) -> "wave "/1
  Discrete Derivative/1 -> Display/1

== system Acquisition_from_autosave/Tracking Loop/Tracking Loops/Tracking Loop5/Oscillator ==
  phase error : Inport
  Acq Freq : Inport  Port=2
  2*pi2 : Constant  Value=2*pi
  2^N2 : Constant  Value=2^16
  Add : Sum
  Counter Free-Running : simulink/Sources/Counter Free-Running  NumBits=15  tsamp=1/32768000
  Divide1 : Product  Inputs=*/
  Divide10 : Product
  Divide8 : Product  Inputs=*/*
  Divide9 : Product  Inputs=***
  Fs2 : Constant  Value=32768000
  IC : InitialCondition  Value=9207000
  MATLAB Function2 : MATLAB Function  TreatAsAtomicUnit=on
  Math Function : Math  Operator=mod  SaturateOnIntegerOverflow=on
  Pulse Generator1 : DiscretePulseGenerator  PulseType=Time based  Period=0.005  PulseWidth=50
  RT2 : RateTransition
  Real-Imag to Complex2 : RealImagToComplex
  Resettable Delay : Delay  DelayLength=1  ExternalReset=Rising  SampleTime=0.001
      settings: InputPortMap=u0,r5
  Sum2 : Sum  Inputs=-+|
  Out1 : Outport
  wires:
  2*pi2/1 -> Divide9/3, Divide10/1
  Sum2/1 -> Divide9/1
  Divide8/1 -> Sum2/2
  2^N2/1 -> Divide10/2, Divide1/2, Divide9/2
  Fs2/1 -> Divide8/2
  Divide10/1 -> Math Function/2
  phase error/1 -> Sum2/1
  Acq Freq/1 -> Divide8/1
  Pulse Generator1/1 -> RT2/1
  MATLAB Function2/1(I) -> Real-Imag to Complex2/1
  MATLAB Function2/2(Q) -> Real-Imag to Complex2/2
  Divide1/1 -> IC/1
  IC/1 -> MATLAB Function2/1(u)
  Resettable Delay/1 -> Add/1
  Math Function/1 -> Resettable Delay/1, Divide1/1
  Add/1 -> Math Function/1
  Divide9/1 -> Add/2
  Real-Imag to Complex2/1 -> Out1/1
  Counter Free-Running/1 -> Divide8/3

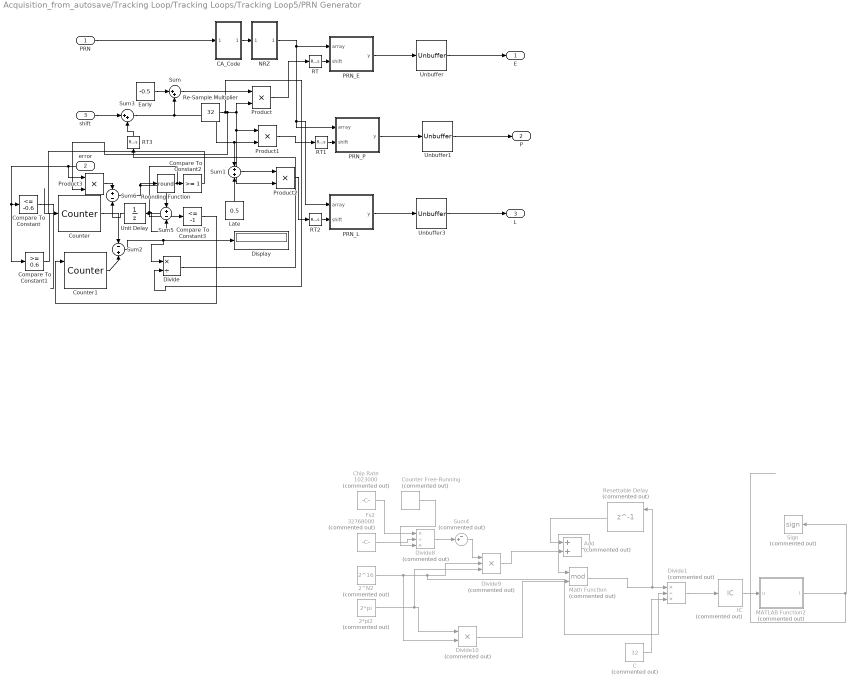
== system Acquisition_from_autosave/Tracking Loop/Tracking Loops/Tracking Loop5/PRN Generator  ==
  PRN : Inport
  error : Inport  Port=2  SampleTime=0.001
  shift : Inport  Port=3
  2*pi2 : Constant  Commented=on  Value=2*pi
  2^N2 : Constant  Commented=on  Value=2^16
  Add : Sum  Commented=on
  C : Constant  Commented=on  Value=32
  "CA_Code " : Subsystem
  Chip Rate : Constant  Commented=on  Value=1023000
  Compare To Constant : simulink/Logic and Bit Operations/Compare To Constant  relop=<=  const=-0.6  OutDataTypeStr=boolean
  Compare To Constant1 : simulink/Logic and Bit Operations/Compare To Constant  relop=>=  const=0.6  OutDataTypeStr=boolean
  Compare To Constant2 : simulink/Logic and Bit Operations/Compare To Constant  relop=>=  const=1  OutDataTypeStr=uint8
  Compare To Constant3 : simulink/Logic and Bit Operations/Compare To Constant  relop=<=  const=-1  OutDataTypeStr=uint8
  Counter : dspswit3/Counter  Direction=Up  CountEvent=Non-zero sample  CounterSize=User defined  MaxCount=255  InitialCount=0  Output=Count  HitValue=32  ResetInput=off  SamplesPerFrame=1  Ts=1  CntDtype=double  HitDtype=Logical
  Counter Free-Running : simulink/Sources/Counter Free-Running  Commented=on  NumBits=15  tsamp=1/32768000
  Counter1 : dspswit3/Counter  Direction=Up  CountEvent=Non-zero sample  CounterSize=User defined  MaxCount=255  InitialCount=0  Output=Count  HitValue=32  ResetInput=on  SamplesPerFrame=1  Ts=1  CntDtype=double  HitDtype=Logical
  Display : Display
  Divide : Product  Inputs=*/
  Divide1 : Product  Commented=on  Inputs=*/*
  Divide10 : Product  Commented=on
  Divide8 : Product  Commented=on  Inputs=*/*
  Divide9 : Product  Commented=on  Inputs=***
  Early : Constant  Value=-0.5
  Fs2 : Constant  Commented=on  Value=32768000
  IC : InitialCondition  Commented=on  Value=1023000
  Late : Constant  Value=0.5
  MATLAB Function2 : MATLAB Function  Commented=on  TreatAsAtomicUnit=on
  Math Function : Math  Commented=on  Operator=mod  SaturateOnIntegerOverflow=on
  NRZ : Subsystem
  PRN_E : MATLAB Function  TreatAsAtomicUnit=on  SystemSampleTime=0.001
  PRN_L : MATLAB Function  TreatAsAtomicUnit=on  SystemSampleTime=0.001
  PRN_P : MATLAB Function  TreatAsAtomicUnit=on  SystemSampleTime=0.001
  Product{,1..3} (4 alike) : Product
  RT : RateTransition  OutPortSampleTime=0.001
  RT1 : RateTransition  OutPortSampleTime=0.001
  RT2 : RateTransition  OutPortSampleTime=0.001
  RT3 : RateTransition
  Re-Sample Multiplier : Constant  Value=32
  Resettable Delay : Delay  Commented=on  DelayLength=1  ExternalReset=Rising  SampleTime=0.001
      settings: InputPortMap=u0,r5
  Rounding Function : Rounding  Operator=round
  Sign : Signum  Commented=on
  Sum : Sum  Inputs=|++
  Sum1 : Sum
  Sum2 : Sum  Inputs=-+
  Sum3 : Sum  Inputs=|++
  Sum4 : Sum  Commented=on  Inputs=-+|
  Sum5 : Sum  Inputs=+-
  Sum6 : Sum  Inputs=+-
  Unbuffer : Unbuffer
  Unbuffer1 : Unbuffer
  Unbuffer3 : Unbuffer
  Unit Delay : UnitDelay  SampleTime=0.001
  E : Outport
  P : Outport  Port=2
  L : Outport  Port=3
  wires:
  Product/1 -> RT/1
  PRN_E/1(y) -> Unbuffer/1
  Product2/1 -> RT2/1
  PRN_L/1(y) -> Unbuffer3/1
  Re-Sample Multiplier/1 -> Divide/2, Product3/2, Product1/1, Product2/2, Product/2
  PRN/1 -> "CA_Code "/1(In1)
  Unbuffer1/1 -> P/1
  Unbuffer3/1 -> L/1
  Early/1 -> Sum/1
  Sum/1 -> Product/1
  Sum3/1 -> Product1/2, Sum1/1, Sum/2
  Sum1/1 -> Product2/1
  PRN_P/1(y) -> Unbuffer1/1
  error/1 -> Product3/1, Compare To Constant1/1, Compare To Constant/1
  Counter/1 -> Sum2/1
  Counter1/1 -> Sum2/2
  Sum2/1 -> Divide/1, Display/1
  shift/1 -> Sum3/1
  RT/1 -> PRN_E/2(shift)
  RT1/1 -> PRN_P/2(shift)
  RT2/1 -> PRN_L/2(shift)
  Late/1 -> Sum1/2
  "CA_Code "/1(Out1) -> NRZ/1(In1)
  Unbuffer/1 -> E/1
  NRZ/1(Out1) -> PRN_E/1(array), PRN_L/1(array), PRN_P/1(array)
  Product1/1 -> RT1/1
  RT3/1 -> Sum3/2
  Compare To Constant1/1 -> ?
  Compare To Constant/1 -> ?
  MATLAB Function2/1(I) -> Sign/1
  Divide8/1 -> Sum4/2
  C/1 -> Divide1/3
  2^N2/1 -> Divide10/2, Divide1/2, Divide9/2
  Fs2/1 -> Divide8/2
  2*pi2/1 -> Divide9/3, Divide10/1
  Sum4/1 -> Divide9/1
  IC/1 -> MATLAB Function2/1(u)
  Divide10/1 -> Math Function/2
  Chip Rate/1 -> Divide8/1
  Resettable Delay/1 -> Add/1
  Divide1/1 -> IC/1
  Divide9/1 -> Add/2
  Counter Free-Running/1 -> Divide8/3
  Add/1 -> Math Function/1
  Math Function/1 -> Resettable Delay/1, Divide1/1
  Compare To Constant2/1 -> Counter/1
  Compare To Constant3/1 -> Counter1/1
  Divide/1 -> RT3/1
  Rounding Function/1 -> Sum5/2, Compare To Constant3/1, Compare To Constant2/1
  Product3/1 -> Sum6/1
  Sum5/1 -> Unit Delay/1
  Sum6/1 -> Sum5/1, Rounding Function/1
  Unit Delay/1 -> Sum6/2

== system Acquisition_from_autosave/Tracking Loop/Tracking Loops/Tracking Loop1/Carrier Filter/Filter Parameters ==
  BW : Constant  Value=25
  Constant : Constant  Value=8
  Constant1 : Constant  Value=4
  Constant2 : Constant
  Constant3 : Constant  Value=2
  Damping : Constant  Value=0.707
  Divide : Product  Inputs=*/
  Gain 1 : Product  Inputs=***/
  Gain 2 : Product  Inputs=**/
  K : Constant
  Product : Product  Inputs=3
  Product1 : Product  Inputs=3
  Sum : Sum  Inputs=|++
  K1 : Outport
  K2 : Outport  Port=2
  wires:
  Damping/1 -> Gain 1/3, Product1/2, Product1/1, Product/3
  K/1 -> Gain 2/3, Gain 1/4
  BW/1 -> Product/2
  Constant/1 -> Product/1
  Product/1 -> Divide/1
  Constant1/1 -> Product1/3
  Constant2/1 -> Sum/1
  Product1/1 -> Sum/2
  Sum/1 -> Divide/2
  Divide/1 -> Gain 2/2, Gain 2/1, Gain 1/1
  Constant3/1 -> Gain 1/2
  Gain 1/1 -> K1/1
  Gain 2/1 -> K2/1

== system Acquisition_from_autosave/Tracking Loop/Tracking Loops/Tracking Loop1/Carrier Filter/Subsystem ==
  BW : Constant  Value=30
  C1 : Subsystem
  C2 : Subsystem
  Constant1 : Constant  Value=8
  Constant2 : Constant  Value=4
  Constant4 : Constant
  Damping : Constant  Value=0.707
  K : Constant  Value=4
  T : Constant  Value=0.001
  Wn : Subsystem
  "K2 " : Outport
  K1 : Outport  Port=2
  wires:
  C1/1(Out1) -> K1/1
  Constant1/1 -> C1/1(In1), Wn/1(In1)
  BW/1 -> Wn/2(In2)
  Damping/1 -> C1/2(In2), C1/3(In3), Wn/3(In3), C2/3(In3), C2/2(In2)
  Constant2/1 -> C2/5(In5), C1/7(In7), C2/6(In6), C2/7(In7), C1/8(In8), Wn/4(In4)
  Constant4/1 -> Wn/5(In5)
  T/1 -> C1/4(In4), C1/5(In5), C1/6(In6), C2/4(In4)
  Wn/1(Out1) -> C1/10(In10), C2/8(In8), C1/9(In9)
  C2/1(Out1) -> "K2 "/1
  K/1 -> C1/11(In11), C2/1(In1)

== system Acquisition_from_autosave/Tracking Loop/Tracking Loops/Tracking Loop1/Filter/Filter Parameters ==
  BW : Constant  Value=25
  Constant : Constant  Value=8
  Constant1 : Constant  Value=4
  Constant2 : Constant
  Constant3 : Constant  Value=2
  Damping : Constant  Value=0.707
  Divide : Product  Inputs=*/
  Gain 1 : Product  Inputs=***/
  Gain 2 : Product  Inputs=**/
  K : Constant
  Product : Product  Inputs=3
  Product1 : Product  Inputs=3
  Sum : Sum  Inputs=|++
  K1 : Outport
  K2 : Outport  Port=2
  wires:
  Damping/1 -> Gain 1/3, Product1/2, Product1/1, Product/3
  K/1 -> Gain 2/3, Gain 1/4
  BW/1 -> Product/2
  Constant/1 -> Product/1
  Product/1 -> Divide/1
  Constant1/1 -> Product1/3
  Constant2/1 -> Sum/1
  Product1/1 -> Sum/2
  Sum/1 -> Divide/2
  Divide/1 -> Gain 2/2, Gain 2/1, Gain 1/1
  Constant3/1 -> Gain 1/2
  Gain 1/1 -> K1/1
  Gain 2/1 -> K2/1

== system Acquisition_from_autosave/Tracking Loop/Tracking Loops/Tracking Loop1/Filter/Subsystem ==
  BW : Constant  Value=30
  C1 : Subsystem
  C2 : Subsystem
  Constant1 : Constant  Value=8
  Constant2 : Constant  Value=4
  Constant4 : Constant
  Damping : Constant  Value=0.707
  K : Constant  Value=4
  T : Constant  Value=0.001
  Wn : Subsystem
  "K2 " : Outport
  K1 : Outport  Port=2
  wires:
  C1/1(Out1) -> K1/1
  Constant1/1 -> C1/1(In1), Wn/1(In1)
  BW/1 -> Wn/2(In2)
  Damping/1 -> C1/2(In2), C1/3(In3), Wn/3(In3), C2/3(In3), C2/2(In2)
  Constant2/1 -> C2/5(In5), C1/7(In7), C2/6(In6), C2/7(In7), C1/8(In8), Wn/4(In4)
  Constant4/1 -> Wn/5(In5)
  T/1 -> C1/4(In4), C1/5(In5), C1/6(In6), C2/4(In4)
  Wn/1(Out1) -> C1/10(In10), C2/8(In8), C1/9(In9)
  C2/1(Out1) -> "K2 "/1
  K/1 -> C1/11(In11), C2/1(In1)

== system Acquisition_from_autosave/Tracking Loop/Tracking Loops/Tracking Loop1/PRN Generator /CA_Code  ==
  In1 : Inport
  CA_Code : MATLAB Function  TreatAsAtomicUnit=on  SystemSampleTime=0.001
  Constant1 : Constant  Value=32
  RT : RateTransition  OutPortSampleTime=0.001
  Reshape : Reshape  OutputDimensionality=Column vector (2-D)
  Out1 : Outport
  wires:
  In1/1 -> RT/1
  CA_Code/1(g) -> Reshape/1
  Constant1/1 -> CA_Code/2(fs)
  Reshape/1 -> Out1/1
  RT/1 -> CA_Code/1(sv)

== system Acquisition_from_autosave/Tracking Loop/Tracking Loops/Tracking Loop1/PRN Generator /NRZ ==
  In1 : Inport
  Constant5 : Constant  Value=2  SampleTime=-1
  Constant6 : Constant  Value=-1
  Product4 : Product
  Sum4 : Sum  Inputs=|++
  Out1 : Outport
  wires:
  Constant6/1 -> Sum4/1
  Sum4/1 -> Out1/1
  Product4/1 -> Sum4/2
  In1/1 -> Product4/2
  Constant5/1 -> Product4/1

== system Acquisition_from_autosave/Tracking Loop/Tracking Loops/Tracking Loop2/Carrier Filter/Filter Parameters ==
  BW : Constant  Value=25
  Constant : Constant  Value=8
  Constant1 : Constant  Value=4
  Constant2 : Constant
  Constant3 : Constant  Value=2
  Damping : Constant  Value=0.707
  Divide : Product  Inputs=*/
  Gain 1 : Product  Inputs=***/
  Gain 2 : Product  Inputs=**/
  K : Constant
  Product : Product  Inputs=3
  Product1 : Product  Inputs=3
  Sum : Sum  Inputs=|++
  K1 : Outport
  K2 : Outport  Port=2
  wires:
  Damping/1 -> Gain 1/3, Product1/2, Product1/1, Product/3
  K/1 -> Gain 2/3, Gain 1/4
  BW/1 -> Product/2
  Constant/1 -> Product/1
  Product/1 -> Divide/1
  Constant1/1 -> Product1/3
  Constant2/1 -> Sum/1
  Product1/1 -> Sum/2
  Sum/1 -> Divide/2
  Divide/1 -> Gain 2/2, Gain 2/1, Gain 1/1
  Constant3/1 -> Gain 1/2
  Gain 1/1 -> K1/1
  Gain 2/1 -> K2/1

== system Acquisition_from_autosave/Tracking Loop/Tracking Loops/Tracking Loop2/Carrier Filter/Subsystem ==
  BW : Constant  Value=30
  C1 : Subsystem
  C2 : Subsystem
  Constant1 : Constant  Value=8
  Constant2 : Constant  Value=4
  Constant4 : Constant
  Damping : Constant  Value=0.707
  K : Constant  Value=4
  T : Constant  Value=0.001
  Wn : Subsystem
  "K2 " : Outport
  K1 : Outport  Port=2
  wires:
  C1/1(Out1) -> K1/1
  Constant1/1 -> C1/1(In1), Wn/1(In1)
  BW/1 -> Wn/2(In2)
  Damping/1 -> C1/2(In2), C1/3(In3), Wn/3(In3), C2/3(In3), C2/2(In2)
  Constant2/1 -> C2/5(In5), C1/7(In7), C2/6(In6), C2/7(In7), C1/8(In8), Wn/4(In4)
  Constant4/1 -> Wn/5(In5)
  T/1 -> C1/4(In4), C1/5(In5), C1/6(In6), C2/4(In4)
  Wn/1(Out1) -> C1/10(In10), C2/8(In8), C1/9(In9)
  C2/1(Out1) -> "K2 "/1
  K/1 -> C1/11(In11), C2/1(In1)

== system Acquisition_from_autosave/Tracking Loop/Tracking Loops/Tracking Loop2/Code Filter/Coeffiecients ==
  BW : Inport
  Zeta : Inport  Port=2
  ts : Inport  Port=3
  Constant1 : Constant  Value=2
  Divide1 : Product  Inputs=**/
  Math Function : Math  Operator=square  SaturateOnIntegerOverflow=on
  Math Function1 : Math  Operator=reciprocal  SaturateOnIntegerOverflow=on
  Wn : Subsystem
  "calc1 " : Subsystem
  calc2 : Product  Inputs=/*
  C1 : Outport
  C2 : Outport  Port=2
  wires:
  BW/1 -> Wn/1(BW)
  Zeta/1 -> Divide1/2, Wn/2(Zeta)
  Math Function/1 -> Math Function1/1
  Constant1/1 -> "calc1 "/1(2), Divide1/1
  Math Function1/1 -> "calc1 "/3(t1), calc2/1
  "calc1 "/1(Out1) -> C1/1
  calc2/1 -> C2/1
  Divide1/1 -> "calc1 "/2(t2)
  Wn/1(Wn) -> Divide1/3, Math Function/1
  ts/1 -> "calc1 "/4(ts), calc2/2

== system Acquisition_from_autosave/Tracking Loop/Tracking Loops/Tracking Loop2/PRN Generator /CA_Code  ==
  In1 : Inport
  CA_Code : MATLAB Function  TreatAsAtomicUnit=on  SystemSampleTime=0.001
  Constant1 : Constant  Value=32
  RT : RateTransition  OutPortSampleTime=0.001
  Reshape : Reshape  OutputDimensionality=Column vector (2-D)
  Out1 : Outport
  wires:
  In1/1 -> RT/1
  CA_Code/1(g) -> Reshape/1
  Constant1/1 -> CA_Code/2(fs)
  Reshape/1 -> Out1/1
  RT/1 -> CA_Code/1(sv)

== system Acquisition_from_autosave/Tracking Loop/Tracking Loops/Tracking Loop2/PRN Generator /NRZ ==
  In1 : Inport
  Constant5 : Constant  Value=2  SampleTime=-1
  Constant6 : Constant  Value=-1
  Product4 : Product
  Sum4 : Sum  Inputs=|++
  Out1 : Outport
  wires:
  Constant6/1 -> Sum4/1
  Sum4/1 -> Out1/1
  Product4/1 -> Sum4/2
  In1/1 -> Product4/2
  Constant5/1 -> Product4/1

== system Acquisition_from_autosave/Tracking Loop/Tracking Loops/Tracking Loop3/Carrier Filter/Filter Parameters ==
  BW : Constant  Value=25
  Constant : Constant  Value=8
  Constant1 : Constant  Value=4
  Constant2 : Constant
  Constant3 : Constant  Value=2
  Damping : Constant  Value=0.707
  Divide : Product  Inputs=*/
  Gain 1 : Product  Inputs=***/
  Gain 2 : Product  Inputs=**/
  K : Constant
  Product : Product  Inputs=3
  Product1 : Product  Inputs=3
  Sum : Sum  Inputs=|++
  K1 : Outport
  K2 : Outport  Port=2
  wires:
  Damping/1 -> Gain 1/3, Product1/2, Product1/1, Product/3
  K/1 -> Gain 2/3, Gain 1/4
  BW/1 -> Product/2
  Constant/1 -> Product/1
  Product/1 -> Divide/1
  Constant1/1 -> Product1/3
  Constant2/1 -> Sum/1
  Product1/1 -> Sum/2
  Sum/1 -> Divide/2
  Divide/1 -> Gain 2/2, Gain 2/1, Gain 1/1
  Constant3/1 -> Gain 1/2
  Gain 1/1 -> K1/1
  Gain 2/1 -> K2/1

== system Acquisition_from_autosave/Tracking Loop/Tracking Loops/Tracking Loop3/Carrier Filter/Subsystem ==
  BW : Constant  Value=30
  C1 : Subsystem
  C2 : Subsystem
  Constant1 : Constant  Value=8
  Constant2 : Constant  Value=4
  Constant4 : Constant
  Damping : Constant  Value=0.707
  K : Constant  Value=4
  T : Constant  Value=0.001
  Wn : Subsystem
  "K2 " : Outport
  K1 : Outport  Port=2
  wires:
  C1/1(Out1) -> K1/1
  Constant1/1 -> C1/1(In1), Wn/1(In1)
  BW/1 -> Wn/2(In2)
  Damping/1 -> C1/2(In2), C1/3(In3), Wn/3(In3), C2/3(In3), C2/2(In2)
  Constant2/1 -> C2/5(In5), C1/7(In7), C2/6(In6), C2/7(In7), C1/8(In8), Wn/4(In4)
  Constant4/1 -> Wn/5(In5)
  T/1 -> C1/4(In4), C1/5(In5), C1/6(In6), C2/4(In4)
  Wn/1(Out1) -> C1/10(In10), C2/8(In8), C1/9(In9)
  C2/1(Out1) -> "K2 "/1
  K/1 -> C1/11(In11), C2/1(In1)
